simulink model "Light_duty_Brushed_DC_Motor_R2020a"  (R2020a)
settings: Solver=VariableStepAuto  StartTime=0.0  StopTime=60*60*8  RelTol=1e-3
undefined symbols (not defined in the file): Rotor_inertia_DC, Torque_Load
libraries: nesl_utility x6, fl_lib x5, ee_lib x4, simulink x1
settings Model: Creator=YXL1108  LastModifiedBy=YXL1108

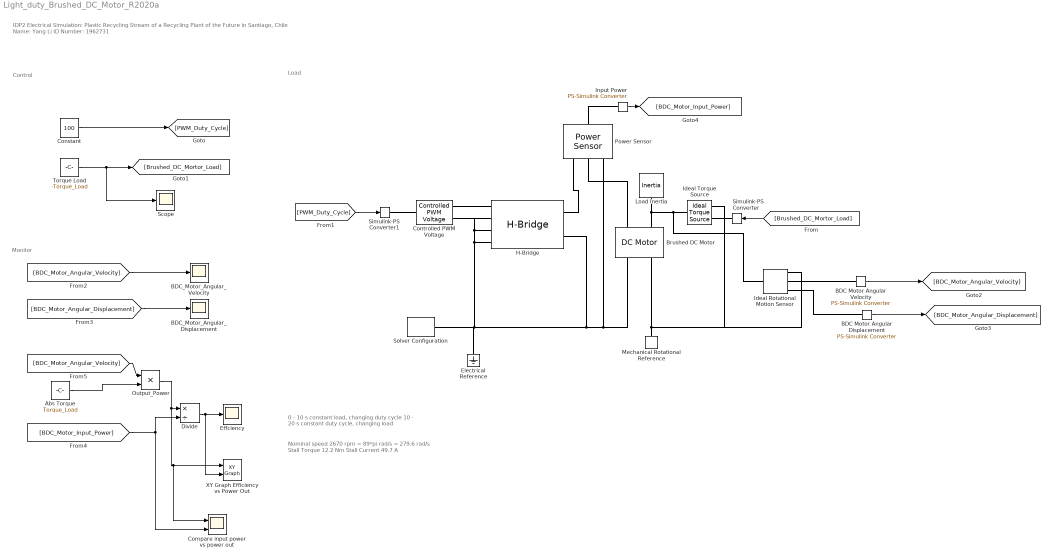
== system Light_duty_Brushed_DC_Motor_R2020a ==
  note: 0 - 10 s constant load, changing duty cycle
      | 10 - 20 s constant duty cycle, changing load
  note: Nominal speed 2670 rpm = 89*pi rad/s = 279.6 rad/s
      | Stall Torque 12.2 Nm
      | Stall Current 49.7 A
  note: Monitor
  note: Control
  note: Load
  note: IDP2 Electrical Simulation: Plastic Recycling Stream of a Recycling Plant of the Future in Santiago, Chile
      | Name: Yang Li
      | ID Number: 1962731
  Abs Torque : Constant  Value=Torque_Load
  BDC Motor Angular Displacement : nesl_utility/PS-Simulink Converter  PhysicalDomain=network_engine_domain  SubClassName=ps_output  LeftPortType=input  RightPortType=output  PseudoPeriodic=off  Frequencies=[]  Unit=inherit  AffineConversion=off
      settings: SourceProductBaseCode=PW,SS
  BDC Motor Angular Velocity : nesl_utility/PS-Simulink Converter  PhysicalDomain=network_engine_domain  SubClassName=ps_output  LeftPortType=input  RightPortType=output  PseudoPeriodic=off  Frequencies=[]  Unit=inherit  AffineConversion=off
      settings: SourceProductBaseCode=PW,SS
  BDC_Motor_Angular_Displacement : Scope
  BDC_Motor_Angular_Velocity : Scope
  Brushed DC Motor : ee_lib/Electromechanical/Brushed Motors/DC Motor  field_option=ee.enum.field_option.pm  Rf=100 Ohm  Lf=1 H  Laf=0.15 H  If0=0 A  parameterization=ee.enum.dcparam_option.torque_speed  Ra=Armature_resistance Ohm  La=Armature_inductance mH  emf_or_torque=ee.enum.emf_or_torque.kv  Kv=Back_emf_constant V/rpm  Ki=6.876e-4 N*m/A  T_stall=Stall_torque mN*m  w_max=No_load_speed rpm  w_rated=15000 rpm  P_rated=0.08 W  V_rated=Rated_DC_supply_voltage V  J=Rotor_inertia_DC g*cm^2  lam_param=ee.enum.lam_param.current  lam=Rotor_damping N*m/(rad/s)  i_noload=No_load_current mA  V_i_noload=Rated_DC_supply_voltage V  speed0=Initial_rotor_speed_DC rpm  alpha=3.93e-3 1/K  Tmeas=25 degC  thermal_mass=100 J/K  initial_temperature=25 degC
      settings: LogSimulationData=on
  Compare input power vs power out : Scope  NumInputPorts=2
  Constant : Constant  Value=100
  Controlled PWM Voltage : ee_lib/Integrated Circuits/Controlled PWM Voltage  F=1000 Hz  TD=0 s  pulse_width_offset=0 s  pulse_min=0 s  Vmin=0 V  Vmax=5 V  Vm=5 V  pwm_or_av=2  event_type=2  sample_time=1e-6 s  u_min=0  u_max=100
      settings: InternalSimscapePortConfiguration="{\"Bottom\":[],\"Left\":[{\"id\":\"u\",\"label\":\"u\",\"type\":\"input\"}],\"Right\":[{\"id\":\"p2\",\"label\":\"PWM\",\"type\":\"foundation.electrical.electrical\"},{\"id\":\"n2\",\"label\":\"REF\",\"type\":\"foundation.electrical.electrical\"}],\"Top\":[]}"
  Divide : Product  Inputs=*/
  Effciency : Scope
  Electrical Reference : fl_lib/Electrical/Electrical Elements/Electrical Reference
  H-Bridge : ee_lib/Semiconductors & Converters/Converters/H-Bridge  supply_ports=ee.enum.supply_ports.hidesupply  Venable=2.5 V  Vmax=5.0 V  Vreverse=2.5 V  Vbrake=2.5 V  Vm=70 V  pwm_or_av=ee.enum.pwm_or_av.averaged  regenerative_braking_mode=ee.enum.converters.regenerative_braking_mode.always_enabled  discontinuous=ee.enum.current_profile.continuous  freewheeling_mode=ee.enum.converters.freewheeling_mode.one_switch_one_diode  Ron=0.1 Ohm  Don=0.05 Ohm  Goff=1e-6 S  Rload=10 Ohm  Lload=1e-5 H  F=10 kHz  thermal_mass=100 J/K  initial_temperature=298.15 K  Ron2=0.1 Ohm  Don2=0.05 Ohm  Tmeas=298.15 K  Tmeas2=398.15 K
  Ideal Rotational Motion Sensor : fl_lib/Mechanical/Mechanical Sensors/Ideal Rotational Motion Sensor  wrap_angle=simscape.enum.onoff.off  offset=0 rad
  Ideal Torque Source : fl_lib/Mechanical/Mechanical Sources/Ideal Torque Source
  Input Power : nesl_utility/PS-Simulink Converter  PhysicalDomain=network_engine_domain  SubClassName=ps_output  LeftPortType=input  RightPortType=output  PseudoPeriodic=off  Frequencies=[]  Unit=inherit  AffineConversion=off
      settings: SourceProductBaseCode=PW,SS
  Load Inertia : fl_lib/Mechanical/Rotational Elements/Inertia  inertia=0.01 kg*m^2  w_specify=off  w_priority=High  w=0 rad/s  w_nominal_specify=off  w_nominal_unit=rad/s  w_nominal_value=1  t_specify=off  t_priority=None  t=0 N*m  t_nominal_specify=off  t_nominal_unit=N*m  t_nominal_value=1
  Mechanical Rotational Reference : fl_lib/Mechanical/Rotational Elements/Mechanical Rotational Reference
  Output_Power : Product
  Power Sensor : ee_lib/Sensors & Transducers/Power Sensor  measurement_type=1  averaging_period=1e-4 s
      settings: SourceProductBaseCode=PS
  Scope : Scope
  Simulink-PS Converter : nesl_utility/Simulink-PS Converter  PhysicalDomain=network_engine_domain  SubClassName=ps_input  LeftPortType=input  RightPortType=output  PseudoPeriodic=off  Frequencies=[]  NoiseDistribution=none  NoiseParameters=[]  Unit=1  AffineConversion=off  FilteringAndDerivatives=provide  SimscapeFilterOrder=1  InputFilterTimeConstant=0.001  UdotUserProvided=0
      settings: SourceProductBaseCode=PW,SS
  Simulink-PS Converter1 : nesl_utility/Simulink-PS Converter  PhysicalDomain=network_engine_domain  SubClassName=ps_input  LeftPortType=input  RightPortType=output  PseudoPeriodic=off  Frequencies=[]  NoiseDistribution=none  NoiseParameters=[]  Unit=1  AffineConversion=off  FilteringAndDerivatives=provide  SimscapeFilterOrder=1  InputFilterTimeConstant=0.001  UdotUserProvided=0
      settings: SourceProductBaseCode=PW,SS
  Solver Configuration : nesl_utility/Solver Configuration  PhysicalDomain=network_engine_domain  SubClassName=solver  LeftPortType=input  RightPortType=generic  Tones=[]  Harmonics=[]  SimulateNoise=off  Profile=off  UseLocalSampling=off  EnableSwitchedLinearOptims=on  FrequencyDomain=off  UseCCode=off  RelTol=0.001  AbsTol=1e-06  MinStep=1e-09  ToWorkspace=off  RevertToSquareIcSolve=off  NumHomotopyIterations=100  PhasorMode=off  PhasorModeNumHarmonics=1  DoDC=off  ResidualTolerance=1e-09  UseLocalSolver=off  LocalSolverChoice=NE_BACKWARD_EULER_ADVANCER  LocalSolverSampleTime=0.001  DoFixedCost=off  MaxNonlinIter=3  MaxModeIter=2  LinearAlgebra=auto  EquationFormulation=NE_TIME_EF  DelaysMemoryBudget=1024  AutomaticFiltering=on  FilteringTimeConstant=0.001  PartitionStorageMethod=AS_NEEDED  PartitionMemoryBudget=1024  PartitionMethod=ROBUST
      settings: SourceProductBaseCode=PW,SS
  Torque Load : Constant  Value=-Torque_Load
  XY Graph Efficiency vs Power Out : simulink/Sinks/XY Graph  xmin=0  xmax=300  ymin=0  ymax=1  st=-1
  wires:
  [Brushed_DC_Mortor_Load] -> Simulink-PS Converter/1
  [PWM_Duty_Cycle] -> Simulink-PS Converter1/1
  Torque Load/1 -> Scope/1, [Brushed_DC_Mortor_Load]
  BDC Motor Angular Velocity/1 -> [BDC_Motor_Angular_Velocity]
  BDC Motor Angular Displacement/1 -> [BDC_Motor_Angular_Displacement]
  [BDC_Motor_Angular_Velocity] -> BDC_Motor_Angular_Velocity/1
  [BDC_Motor_Angular_Displacement] -> BDC_Motor_Angular_Displacement/1
  Constant/1 -> [PWM_Duty_Cycle]
  Input Power/1 -> [BDC_Motor_Input_Power]
  [BDC_Motor_Angular_Velocity] -> Output_Power/1
  Abs Torque/1 -> Output_Power/2
  Output_Power/1 -> Compare input power vs power out/1, XY Graph Efficiency vs Power Out/1, Divide/1
  [BDC_Motor_Input_Power] -> Compare input power vs power out/2, Divide/2
  Divide/1 -> XY Graph Efficiency vs Power Out/2, Effciency/1
  connections:
  H-Bridge/LConn1 -- Controlled PWM Voltage/RConn1
  Brushed DC Motor/RConn1 -- H-Bridge/RConn2 -- Solver Configuration/RConn1 -- Electrical Reference/LConn1 -- H-Bridge/LConn4 -- H-Bridge/LConn3 -- H-Bridge/LConn2 -- Controlled PWM Voltage/RConn2 -- Power Sensor/LConn3
  Brushed DC Motor/RConn2 -- Ideal Rotational Motion Sensor/RConn1 -- Ideal Torque Source/RConn2 -- Mechanical Rotational Reference/LConn1
  Brushed DC Motor/LConn2 -- Ideal Rotational Motion Sensor/LConn1 -- Ideal Torque Source/LConn1 -- Load Inertia/LConn1
  Simulink-PS Converter/RConn1 -- Ideal Torque Source/RConn1
  Simulink-PS Converter1/RConn1 -- Controlled PWM Voltage/LConn1
  Ideal Rotational Motion Sensor/RConn2 -- BDC Motor Angular Velocity/LConn1
  BDC Motor Angular Displacement/LConn1 -- Ideal Rotational Motion Sensor/RConn3
  H-Bridge/RConn1 -- Power Sensor/LConn1
  Brushed DC Motor/LConn1 -- Power Sensor/LConn2
  Input Power/LConn1 -- Power Sensor/RConn1
